simulink model "NoPainNoCrane_Hardware"  (R2016a)
settings: Solver=ode5  StartTime=0.0  StopTime=59.6965  FixedStep=0.01  RelTol=1e-3
model workspace: external: MAT-File workspace.mat (data not in the file)
values from neighbouring files (symbols this model uses):
  AngleDX = 0    [RunHWModel.m]    (also in simSetup.m; workspace.mat)
  AngleDY = AngleDX    (= 0)    [RunHWModel.m]    (also in simSetup.m; workspace.mat)
  AngleIX = 0    [RunHWModel.m]    (also in simSetup.m; workspace.mat)
  AngleIY = AngleIX    (= 0)    [RunHWModel.m]    (also in simSetup.m; workspace.mat)
  AnglePX = 2.0    (= 2)    [RunHWModel.m]    (also in simSetup.m; workspace.mat)
  AnglePY = AnglePX    (= 2)    [RunHWModel.m]    (also in simSetup.m; workspace.mat)
  DC1x = 0.1    [RunHWModel.m]    (also in simSetup.m; workspace.mat)
  DC1y = DC1x    (= 0.1)    [RunHWModel.m]    (also in simSetup.m; workspace.mat)
  IC1x = 0.9    [RunHWModel.m]    (also in simSetup.m; workspace.mat)
  IC1y = IC1x    (= 0.9)    [RunHWModel.m]    (also in simSetup.m; workspace.mat)
  PC1x = 4.7    [RunHWModel.m]    (also in simSetup.m; workspace.mat)
  PC1y = PC1x    (= 4.7)    [RunHWModel.m]    (also in simSetup.m; workspace.mat)
  Ts = 1/20    (= 0.05)    [setup.m]    (also in workspace.mat)
  waypoints = [waypoints is_target]    [path_planning.m]    (also in workspace.mat = [0 1 4 16 20 20 0 2 5 6 10 20 ... (30 elements, 6x5)])
  xRange = [0 0.52]    [workspace.mat]
  yRange = [0 0.62]    [workspace.mat]
undefined symbols (not defined in the file or in its folder): Crane3D_RangeBit, Crane3D_ScaleCoeff
undefined symbols (not defined in the file): RTDAC4PCIBaseAddress
libraries: simulink x4
settings Model: SimulationMode=external  ExtModeTrigDuration=10000  Creator=The MathWorks Inc.  LastModifiedBy=mc1713
settings DataIOCC: SaveFormat=StructureWithTime  SignalLoggingSaveFormat=ModelDataLogs  SignalLoggingName=logsOut
settings OptimizationCC: ExpressionDepthLimit=2147483647  InitFltsAndDblsToZero=on  EfficientMapNaN2IntZero=off
settings DebuggingCC: UnderspecifiedInitializationDetection=Classic  MergeDetectMultiDrivingBlocksExec=none  SignalResolutionControl=TryResolveAllWithWarning  FcnCallInpInsideContextMsg=EnableAllAsWarning  StateNameClashWarn=warning
settings HardwareCC: ProdBitPerLong=64  ProdLargestAtomicFloat=None  ProdHWDeviceType=Intel->x86-64  TargetBitPerLong=64  TargetBitPerPointer=64  TargetIntDivRoundTo=Zero  TargetEndianess=LittleEndian  TargetWordSize=64  TargetHWDeviceType=Intel->x86-64
settings ModelReferenceCC: UpdateModelReferenceTargets=Force  PropagateSignalLabelsOutOfModel=off
settings RTWCC: SystemTargetFile=sldrt.tlc  TemplateMakefile=sldrt.tmf  Description=Simulink Desktop Real-Time  RTWCompilerOptimization=on
settings CodeAppCC: MaxIdLength=95
settings TargetCC: TargetPreCompLibLocation=C:\matlab\R2016a\toolbox\sldrt\lib\win64  GeneratePreprocessorConditionals=Use local settings
settings ConfigComp: CovSFcnEnable=off

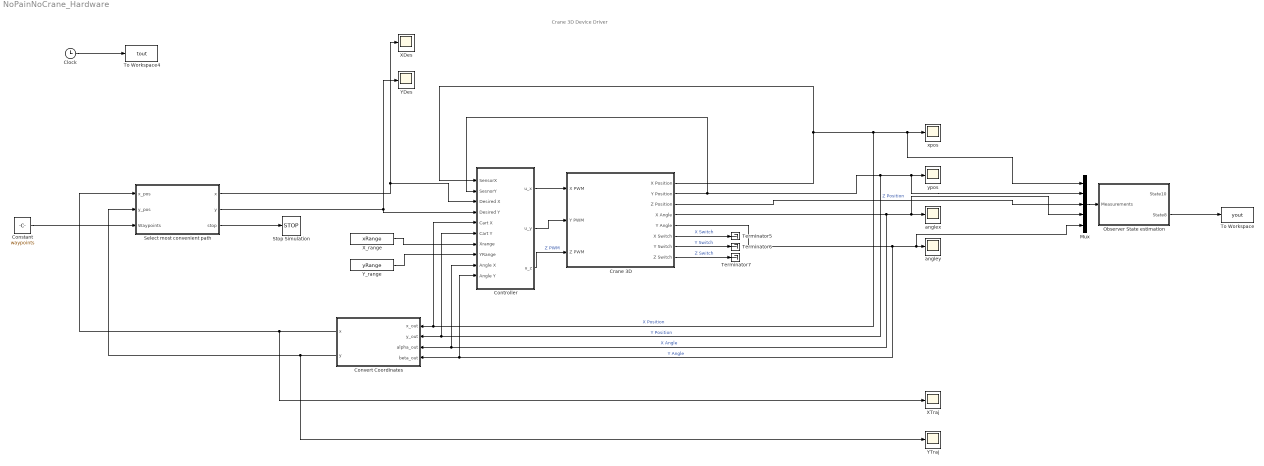
== system NoPainNoCrane_Hardware ==
  note: Crane 3D Device Driver
  Clock : Clock
  Constant : Constant  Value=waypoints
  Controller : Subsystem
  Convert Coordinates : MATLAB Function  TreatAsAtomicUnit=on
  Crane 3D : Subsystem  mask{BaseAddress=RTDAC4PCIBaseAddress, T0=0.01}
      mask prompts: BaseAddress "Base Address:"; T0 "Samping Period:"
      mask Display: image(imread('crane.jpeg'))
  Mux : Mux  Inputs=5
  Observer State estimation : Subsystem
  Select most convenient path : MATLAB Function  TreatAsAtomicUnit=on
  Stop Simulation : Stop
  Terminator5 : Terminator
  Terminator6 : Terminator
  Terminator7 : Terminator
  To Workspace : ToWorkspace  VariableName=yout  SaveFormat=Structure With Time  SampleTime=-1
  To Workspace4 : ToWorkspace  VariableName=tout  SaveFormat=Structure With Time  SampleTime=-1
  XDes : Scope
  XTraj : Scope
  X_range : Constant  Value=xRange
  YDes : Scope
  YTraj : Scope
  "Y_range " : Constant  Value=yRange
  anglex : Scope
  angley : Scope
  xpos : Scope
  ypos : Scope
  wires:
  Crane 3D/6(X Switch) -> Terminator5/1  "X Switch"
  Crane 3D/7(Y Switch) -> Terminator6/1  "Y Switch"
  Crane 3D/8(Z Switch) -> Terminator7/1  "Z Switch"
  Crane 3D/1(X Position) -> Controller/5(Cart X), Convert Coordinates/1(x_out), Mux/1, xpos/1, Controller/1(SensorX)  "X Position"
  Crane 3D/2(Y Position) -> Controller/2(SesnorY), Controller/6(Cart Y), Convert Coordinates/2(y_out), Mux/2, ypos/1  "Y Position"
  Crane 3D/3(Z Position) -> Mux/3  "Z Position"
  Crane 3D/4(X Angle) -> Controller/9(Angle X), Convert Coordinates/3(alpha_out), Mux/4, anglex/1  "X Angle"
  Crane 3D/5(Y Angle) -> Controller/10(Angle Y), Convert Coordinates/4(beta_out), Mux/5, angley/1  "Y Angle"
  Controller/3(u_z) -> Crane 3D/3(Z PWM)  "Z PWM"
  Clock/1 -> To Workspace4/1
  Convert Coordinates/2(y) -> YTraj/1, Select most convenient path/2(y_pos)
  Convert Coordinates/1(x) -> XTraj/1, Select most convenient path/1(x_pos)
  Controller/2(u_y) -> Crane 3D/2(Y PWM)
  Controller/1(u_x) -> Crane 3D/1(X PWM)
  Constant/1 -> Select most convenient path/3(Waypoints)
  Select most convenient path/1(x) -> XDes/1, Controller/3(Desired X)
  Select most convenient path/2(y) -> Controller/4(Desired Y), YDes/1
  X_range/1 -> Controller/7(Xrange)
  "Y_range "/1 -> Controller/8(YRange)
  Select most convenient path/3(stop) -> Stop Simulation/1
  Mux/1 -> Observer State estimation/1(Measurements)
  Observer State estimation/2(State8) -> To Workspace/1

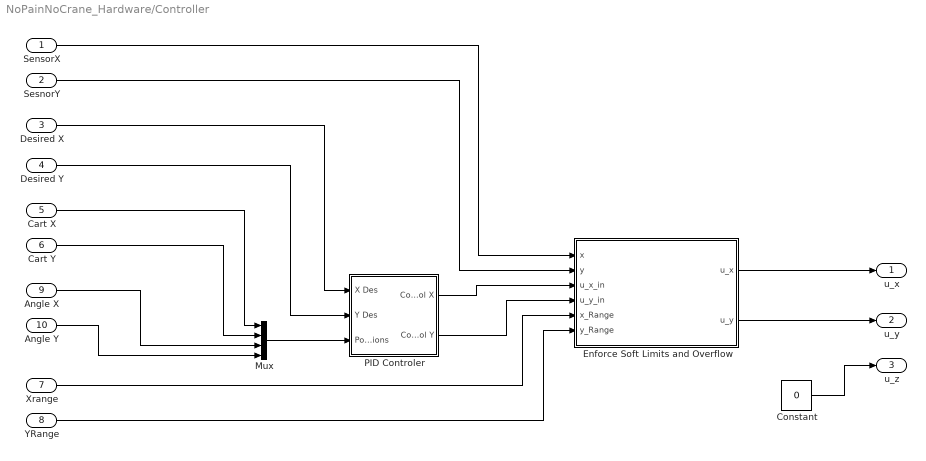
== system NoPainNoCrane_Hardware/Controller ==
  SensorX : Inport
  SesnorY : Inport  Port=2
  Desired X : Inport  Port=3
  Desired Y : Inport  Port=4
  Cart X : Inport  Port=5
  Cart Y : Inport  Port=6
  Xrange : Inport  Port=7
  YRange : Inport  Port=8
  Angle X : Inport  Port=9
  Angle Y : Inport  Port=10
  Constant : Constant  Value=0
  Enforce Soft Limits and Overflow : MATLAB Function  TreatAsAtomicUnit=on
  Mux : Mux
  PID Controler : Subsystem
  u_x : Outport
  u_y : Outport  Port=2
  u_z : Outport  Port=3
  wires:
  Constant/1 -> u_z/1
  Desired X/1 -> PID Controler/1(X Des)
  Desired Y/1 -> PID Controler/2(Y Des)
  Mux/1 -> PID Controler/3(Positions)
  Cart X/1 -> Mux/1
  Cart Y/1 -> Mux/2
  Enforce Soft Limits and Overflow/1(u_x) -> u_x/1
  Enforce Soft Limits and Overflow/2(u_y) -> u_y/1
  PID Controler/1(Control X) -> Enforce Soft Limits and Overflow/3(u_x_in)
  PID Controler/2(Control Y) -> Enforce Soft Limits and Overflow/4(u_y_in)
  Xrange/1 -> Enforce Soft Limits and Overflow/5(x_Range)
  YRange/1 -> Enforce Soft Limits and Overflow/6(y_Range)
  SensorX/1 -> Enforce Soft Limits and Overflow/1(x)
  SesnorY/1 -> Enforce Soft Limits and Overflow/2(y)
  Angle X/1 -> Mux/3
  Angle Y/1 -> Mux/4

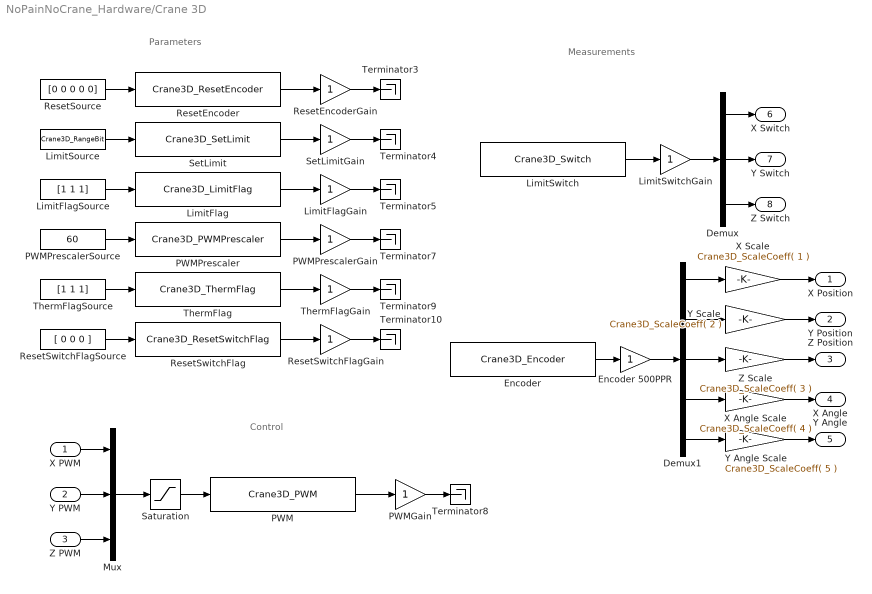
== system NoPainNoCrane_Hardware/Crane 3D ==
  note: Measurements
  note: Control
  note: Parameters
  X PWM : Inport
  Y PWM : Inport  Port=2
  Z PWM : Inport  Port=3
  Demux : Demux  Outputs=3
  Demux1 : Demux  Outputs=5
  Encoder : S-Function  FunctionName=Crane3D_Encoder  Parameters=BaseAddress, T0  SFunctionDeploymentMode=off  EnableBusSupport=off
  Encoder 500PPR : Gain  SaturateOnIntegerOverflow=on  OutDataTypeStr=Inherit: Same as input  ParamDataTypeStr=Inherit: Same as input
  LimitFlag : S-Function  FunctionName=Crane3D_LimitFlag  Parameters=BaseAddress, T0  SFunctionDeploymentMode=off  EnableBusSupport=off
  LimitFlagGain : Gain  SaturateOnIntegerOverflow=on  OutDataTypeStr=Inherit: Same as input  ParamDataTypeStr=Inherit: Same as input
  LimitFlagSource : Constant  Value=[1 1 1]
  LimitSource : Constant  Value=Crane3D_RangeBit
  LimitSwitch : S-Function  FunctionName=Crane3D_Switch  Parameters=BaseAddress, T0  SFunctionDeploymentMode=off  EnableBusSupport=off
  LimitSwitchGain : Gain  SaturateOnIntegerOverflow=on  OutDataTypeStr=Inherit: Same as input  ParamDataTypeStr=Inherit: Same as input
  Mux : Mux  Inputs=3
  PWM : S-Function  FunctionName=Crane3D_PWM  Parameters=BaseAddress, T0  SFunctionDeploymentMode=off  EnableBusSupport=off
  PWMGain : Gain  SaturateOnIntegerOverflow=on  OutDataTypeStr=Inherit: Same as input  ParamDataTypeStr=Inherit: Same as input
  PWMPrescaler : S-Function  FunctionName=Crane3D_PWMPrescaler  Parameters=BaseAddress, T0  SFunctionDeploymentMode=off  EnableBusSupport=off
  PWMPrescalerGain : Gain  SaturateOnIntegerOverflow=on  OutDataTypeStr=Inherit: Same as input  ParamDataTypeStr=Inherit: Same as input
  PWMPrescalerSource : Constant  Value=60
  ResetEncoder : S-Function  FunctionName=Crane3D_ResetEncoder  Parameters=BaseAddress, T0  SFunctionDeploymentMode=off  EnableBusSupport=off
  ResetEncoderGain : Gain  SaturateOnIntegerOverflow=on  OutDataTypeStr=Inherit: Same as input  ParamDataTypeStr=Inherit: Same as input
  ResetSource : Constant  Value=[0 0 0 0 0]
  "ResetSwitchFlag " : S-Function  FunctionName=Crane3D_ResetSwitchFlag  Parameters=BaseAddress, T0  SFunctionDeploymentMode=off  EnableBusSupport=off
  ResetSwitchFlagGain : Gain  SaturateOnIntegerOverflow=on  OutDataTypeStr=Inherit: Same as input  ParamDataTypeStr=Inherit: Same as input
  ResetSwitchFlagSource : Constant  Value=[ 0 0 0 ]
  Saturation : Saturate  UpperLimit=1  LowerLimit=-1
  SetLimit : S-Function  FunctionName=Crane3D_SetLimit  Parameters=BaseAddress, T0  SFunctionDeploymentMode=off  EnableBusSupport=off
  SetLimitGain : Gain  SaturateOnIntegerOverflow=on  OutDataTypeStr=Inherit: Same as input  ParamDataTypeStr=Inherit: Same as input
  Terminator{3..5,7..10} (7 alike) : Terminator
  "ThermFlag " : S-Function  FunctionName=Crane3D_ThermFlag  Parameters=BaseAddress, T0  SFunctionDeploymentMode=off  EnableBusSupport=off
  ThermFlagGain : Gain  SaturateOnIntegerOverflow=on  OutDataTypeStr=Inherit: Same as input  ParamDataTypeStr=Inherit: Same as input
  ThermFlagSource : Constant  Value=[1 1 1]
  X Angle Scale : Gain  Gain=Crane3D_ScaleCoeff( 4 )  OutDataTypeStr=Inherit: Same as input  ParamDataTypeStr=Inherit: Same as input
  X Scale : Gain  Gain=Crane3D_ScaleCoeff( 1 )  OutDataTypeStr=Inherit: Same as input  ParamDataTypeStr=Inherit: Same as input
  Y Angle Scale : Gain  Gain=Crane3D_ScaleCoeff( 5 )  OutDataTypeStr=Inherit: Same as input  ParamDataTypeStr=Inherit: Same as input
  Y Scale : Gain  Gain=Crane3D_ScaleCoeff( 2 )  OutDataTypeStr=Inherit: Same as input  ParamDataTypeStr=Inherit: Same as input
  Z Scale : Gain  Gain=Crane3D_ScaleCoeff( 3 )  OutDataTypeStr=Inherit: Same as input  ParamDataTypeStr=Inherit: Same as input
  X Position : Outport  InitialOutput=0
  Y Position : Outport  Port=2  InitialOutput=0
  Z Position : Outport  Port=3  InitialOutput=0
  X Angle : Outport  Port=4  InitialOutput=0
  Y Angle : Outport  Port=5  InitialOutput=0
  X Switch : Outport  Port=6  InitialOutput=0
  Y Switch : Outport  Port=7  InitialOutput=0
  Z Switch : Outport  Port=8  InitialOutput=0
  wires:
  Demux1/1 -> X Scale/1
  Demux1/2 -> Y Scale/1
  Demux1/3 -> Z Scale/1
  Demux1/4 -> X Angle Scale/1
  Demux1/5 -> Y Angle Scale/1
  X Angle Scale/1 -> X Angle/1
  Y Angle Scale/1 -> Y Angle/1
  Y Scale/1 -> Y Position/1
  X Scale/1 -> X Position/1
  Z Scale/1 -> Z Position/1
  Demux/3 -> Z Switch/1
  Demux/2 -> Y Switch/1
  Demux/1 -> X Switch/1
  LimitSwitchGain/1 -> Demux/1
  LimitSwitch/1 -> LimitSwitchGain/1
  X PWM/1 -> Mux/1
  Y PWM/1 -> Mux/2
  Z PWM/1 -> Mux/3
  ResetSwitchFlagGain/1 -> Terminator10/1
  ThermFlagGain/1 -> Terminator9/1
  PWMPrescalerGain/1 -> Terminator7/1
  LimitFlagGain/1 -> Terminator5/1
  SetLimitGain/1 -> Terminator4/1
  ResetEncoderGain/1 -> Terminator3/1
  ResetSwitchFlagSource/1 -> "ResetSwitchFlag "/1
  ThermFlagSource/1 -> "ThermFlag "/1
  PWMPrescalerSource/1 -> PWMPrescaler/1
  LimitFlagSource/1 -> LimitFlag/1
  LimitSource/1 -> SetLimit/1
  ResetSource/1 -> ResetEncoder/1
  "ResetSwitchFlag "/1 -> ResetSwitchFlagGain/1
  "ThermFlag "/1 -> ThermFlagGain/1
  PWMPrescaler/1 -> PWMPrescalerGain/1
  LimitFlag/1 -> LimitFlagGain/1
  SetLimit/1 -> SetLimitGain/1
  ResetEncoder/1 -> ResetEncoderGain/1
  PWMGain/1 -> Terminator8/1
  PWM/1 -> PWMGain/1
  Mux/1 -> Saturation/1
  Saturation/1 -> PWM/1
  Encoder/1 -> Encoder 500PPR/1
  Encoder 500PPR/1 -> Demux1/1

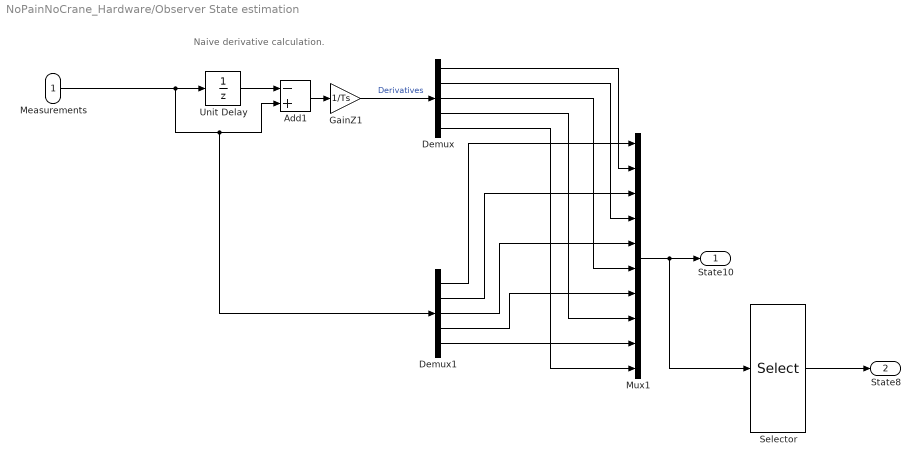
== system NoPainNoCrane_Hardware/Observer State estimation ==
  note: Naive derivative calculation.
  Measurements : Inport
  Add1 : Sum  Inputs=-+
  Demux : Demux  Outputs=5
  Demux1 : Demux  Outputs=5
  GainZ1 : Gain  Gain=1/Ts  SaturateOnIntegerOverflow=on  OutDataTypeStr=Inherit: Same as input  ParamDataTypeStr=Inherit: Same as input
  Mux1 : Mux  Inputs=10
  Selector : Selector  InputPortWidth=10  IndexOptions=Index vector (dialog)  Indices=[1:4 7:10]  OutputSizes=1
  Unit Delay : UnitDelay  InitialCondition="[0.26 0.32 0.3  0 0]"  SampleTime=-1
  State10 : Outport
  State8 : Outport  Port=2
  wires:
  Unit Delay/1 -> Add1/1
  Add1/1 -> GainZ1/1
  Measurements/1 -> Demux1/1, Add1/2, Unit Delay/1
  GainZ1/1 -> Demux/1  "Derivatives"
  Mux1/1 -> Selector/1, State10/1
  Demux1/1 -> Mux1/1
  Demux/1 -> Mux1/2
  Demux1/2 -> Mux1/3
  Demux1/3 -> Mux1/5
  Demux1/4 -> Mux1/7
  Demux1/5 -> Mux1/9
  Demux/2 -> Mux1/4
  Demux/3 -> Mux1/6
  Demux/4 -> Mux1/8
  Demux/5 -> Mux1/10
  Selector/1 -> State8/1

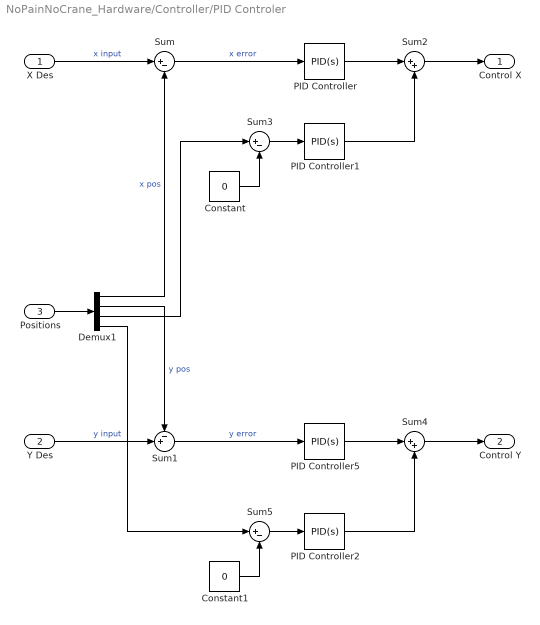
== system NoPainNoCrane_Hardware/Controller/PID Controler ==
  X Des : Inport
  Y Des : Inport  Port=2
  Positions : Inport  Port=3
  Constant : Constant  Value=0
  Constant1 : Constant  Value=0
  Demux1 : Demux
  PID Controller : simulink/Continuous/PID Controller  Controller=PID  TimeDomain=Continuous-time  SampleTime=-1  IntegratorMethod=Forward Euler  FilterMethod=Forward Euler  Form=Parallel  UseFilter=on  ControllerParametersSource=internal  P=PC1x  I=IC1x  D=DC1x  N=30  InitialConditionSource=internal  InitialConditionForIntegrator=0  InitialConditionForFilter=0  ExternalReset=none  LimitOutput=off  UpperSaturationLimit=inf  LowerSaturationLimit=-inf  LinearizeAsGain=on  AntiWindupMode=none  Kb=1  TrackingMode=off  Kt=1  PParamMin=[]  PParamMax=[]  IParamMin=[]  IParamMax=[]  DParamMin=[]  DParamMax=[]  NParamMin=[]  NParamMax=[]  KbParamMin=[]  KbParamMax=[]  KtParamMin=[]  KtParamMax=[]  POutMin=[]  POutMax=[]  IOutMin=[]  IOutMax=[]  DOutMin=[]  DOutMax=[]  NOutMin=[]  NOutMax=[]  KbOutMin=[]  KbOutMax=[]  KtOutMin=[]  KtOutMax=[]  IntegratorOutMin=[]  IntegratorOutMax=[]  FilterOutMin=[]  FilterOutMax=[]  SumOutMin=[]  SumOutMax=[]  SumI1OutMin=[]  SumI1OutMax=[]  SumI2OutMin=[]  SumI2OutMax=[]  SumI3OutMin=[]  SumI3OutMax=[]  SumDOutMin=[]  SumDOutMax=[]  SaturationOutMin=[]  SaturationOutMax=[]  IntegratorContinuousStateAttributes=''  IntegratorStateMustResolveToSignalObject=off  IntegratorRTWStateStorageClass=Auto  FilterContinuousStateAttributes=''  FilterStateMustResolveToSignalObject=off  FilterRTWStateStorageClass=Auto  DifferentiatorICPrevScaledInput=0  DifferentiatorOutMin=[]  DifferentiatorOutMax=[]
  PID Controller1 : simulink/Continuous/PID Controller  Controller=PID  TimeDomain=Continuous-time  SampleTime=-1  IntegratorMethod=Forward Euler  FilterMethod=Forward Euler  Form=Parallel  UseFilter=on  ControllerParametersSource=internal  P=AnglePX  I=AngleIX  D=AngleDX  N=30  InitialConditionSource=internal  InitialConditionForIntegrator=0  InitialConditionForFilter=0  ExternalReset=none  LimitOutput=off  UpperSaturationLimit=inf  LowerSaturationLimit=-inf  LinearizeAsGain=on  AntiWindupMode=none  Kb=1  TrackingMode=off  Kt=1  PParamMin=[]  PParamMax=[]  IParamMin=[]  IParamMax=[]  DParamMin=[]  DParamMax=[]  NParamMin=[]  NParamMax=[]  KbParamMin=[]  KbParamMax=[]  KtParamMin=[]  KtParamMax=[]  POutMin=[]  POutMax=[]  IOutMin=[]  IOutMax=[]  DOutMin=[]  DOutMax=[]  NOutMin=[]  NOutMax=[]  KbOutMin=[]  KbOutMax=[]  KtOutMin=[]  KtOutMax=[]  IntegratorOutMin=[]  IntegratorOutMax=[]  FilterOutMin=[]  FilterOutMax=[]  SumOutMin=[]  SumOutMax=[]  SumI1OutMin=[]  SumI1OutMax=[]  SumI2OutMin=[]  SumI2OutMax=[]  SumI3OutMin=[]  SumI3OutMax=[]  SumDOutMin=[]  SumDOutMax=[]  SaturationOutMin=[]  SaturationOutMax=[]  IntegratorContinuousStateAttributes=''  IntegratorStateMustResolveToSignalObject=off  IntegratorRTWStateStorageClass=Auto  FilterContinuousStateAttributes=''  FilterStateMustResolveToSignalObject=off  FilterRTWStateStorageClass=Auto  DifferentiatorICPrevScaledInput=0  DifferentiatorOutMin=[]  DifferentiatorOutMax=[]
  PID Controller2 : simulink/Continuous/PID Controller  Controller=PID  TimeDomain=Continuous-time  SampleTime=-1  IntegratorMethod=Forward Euler  FilterMethod=Forward Euler  Form=Parallel  UseFilter=on  ControllerParametersSource=internal  P=AnglePY  I=AngleIY  D=AngleDY  N=30  InitialConditionSource=internal  InitialConditionForIntegrator=0  InitialConditionForFilter=0  ExternalReset=none  LimitOutput=off  UpperSaturationLimit=inf  LowerSaturationLimit=-inf  LinearizeAsGain=on  AntiWindupMode=none  Kb=1  TrackingMode=off  Kt=1  PParamMin=[]  PParamMax=[]  IParamMin=[]  IParamMax=[]  DParamMin=[]  DParamMax=[]  NParamMin=[]  NParamMax=[]  KbParamMin=[]  KbParamMax=[]  KtParamMin=[]  KtParamMax=[]  POutMin=[]  POutMax=[]  IOutMin=[]  IOutMax=[]  DOutMin=[]  DOutMax=[]  NOutMin=[]  NOutMax=[]  KbOutMin=[]  KbOutMax=[]  KtOutMin=[]  KtOutMax=[]  IntegratorOutMin=[]  IntegratorOutMax=[]  FilterOutMin=[]  FilterOutMax=[]  SumOutMin=[]  SumOutMax=[]  SumI1OutMin=[]  SumI1OutMax=[]  SumI2OutMin=[]  SumI2OutMax=[]  SumI3OutMin=[]  SumI3OutMax=[]  SumDOutMin=[]  SumDOutMax=[]  SaturationOutMin=[]  SaturationOutMax=[]  IntegratorContinuousStateAttributes=''  IntegratorStateMustResolveToSignalObject=off  IntegratorRTWStateStorageClass=Auto  FilterContinuousStateAttributes=''  FilterStateMustResolveToSignalObject=off  FilterRTWStateStorageClass=Auto  DifferentiatorICPrevScaledInput=0  DifferentiatorOutMin=[]  DifferentiatorOutMax=[]
  PID Controller5 : simulink/Continuous/PID Controller  Controller=PID  TimeDomain=Continuous-time  SampleTime=-1  IntegratorMethod=Forward Euler  FilterMethod=Forward Euler  Form=Parallel  UseFilter=on  ControllerParametersSource=internal  P=PC1y  I=IC1y  D=DC1y  N=30  InitialConditionSource=internal  InitialConditionForIntegrator=0  InitialConditionForFilter=0  ExternalReset=none  LimitOutput=off  UpperSaturationLimit=inf  LowerSaturationLimit=-inf  LinearizeAsGain=on  AntiWindupMode=none  Kb=1  TrackingMode=off  Kt=1  PParamMin=[]  PParamMax=[]  IParamMin=[]  IParamMax=[]  DParamMin=[]  DParamMax=[]  NParamMin=[]  NParamMax=[]  KbParamMin=[]  KbParamMax=[]  KtParamMin=[]  KtParamMax=[]  POutMin=[]  POutMax=[]  IOutMin=[]  IOutMax=[]  DOutMin=[]  DOutMax=[]  NOutMin=[]  NOutMax=[]  KbOutMin=[]  KbOutMax=[]  KtOutMin=[]  KtOutMax=[]  IntegratorOutMin=[]  IntegratorOutMax=[]  FilterOutMin=[]  FilterOutMax=[]  SumOutMin=[]  SumOutMax=[]  SumI1OutMin=[]  SumI1OutMax=[]  SumI2OutMin=[]  SumI2OutMax=[]  SumI3OutMin=[]  SumI3OutMax=[]  SumDOutMin=[]  SumDOutMax=[]  SaturationOutMin=[]  SaturationOutMax=[]  IntegratorContinuousStateAttributes=''  IntegratorStateMustResolveToSignalObject=off  IntegratorRTWStateStorageClass=Auto  FilterContinuousStateAttributes=''  FilterStateMustResolveToSignalObject=off  FilterRTWStateStorageClass=Auto  DifferentiatorICPrevScaledInput=0  DifferentiatorOutMin=[]  DifferentiatorOutMax=[]
  Sum : Sum  Inputs=|+-
  Sum1 : Sum  Inputs=-+|
  Sum2 : Sum  Inputs=|++
  Sum3 : Sum  Inputs=|+-
  Sum4 : Sum  Inputs=|++
  Sum5 : Sum  Inputs=|+-
  Control X : Outport
  Control Y : Outport  Port=2
  wires:
  Demux1/1 -> Sum/2  "x pos"
  X Des/1 -> Sum/1  "x input"
  Sum/1 -> PID Controller/1  "x error"
  Demux1/2 -> Sum1/1  "y pos"
  Y Des/1 -> Sum1/2  "y input"
  Positions/1 -> Demux1/1
  Sum1/1 -> PID Controller5/1  "y error"
  PID Controller/1 -> Sum2/1
  PID Controller1/1 -> Sum2/2
  Sum3/1 -> PID Controller1/1
  Demux1/3 -> Sum3/1
  Constant/1 -> Sum3/2
  Sum2/1 -> Control X/1
  PID Controller5/1 -> Sum4/1
  Sum4/1 -> Control Y/1
  PID Controller2/1 -> Sum4/2
  Sum5/1 -> PID Controller2/1
  Constant1/1 -> Sum5/2
  Demux1/4 -> Sum5/1

== matlab function NoPainNoCrane_Hardware/Controller/Enforce Soft Limits and Overflow ==
  data: x input; u_x output; y input; u_x_in input; u_y_in input; x_Range input; y_Range input; u_y output
function [u_x, u_y] = fcn(x, y, u_x_in, u_y_in, x_Range, y_Range)

buff_up = 0.08;
buff_low = 0.08;
u_x = u_x_in;
u_y = u_y_in;

% Deal with overflow - may not be the most appropriate place
if(x > 10 || x < -10)
   x = 0;
end
if (y > 10 || y < -10)
   y = 0;
end

% Put in place soft boundaries on the borders
if (x > (x_Range(2)-buff_up))
    u_x = min(u_x_in,0);
end

if (x < (x_Range(1)+buff_low))
    u_x = max(u_x_in,0);
end


if (y > (y_Range(2)-buff_up))
    u_y = min(u_y_in,0);
end

if (y < (y_Range(1)+buff_low))
    u_y = max(u_y_in,0);
end


end

== matlab function NoPainNoCrane_Hardware/Select most convenient path ==
  data: x output; y output; x_pos input; y_pos input; Waypoints input; stop output
function [x,y, stop] = Path_Selector(x_pos, y_pos, Waypoints)
persistent WP_Index

if isempty(WP_Index)
    WP_Index = 1;
end

%% Random default values - dont touch
x = 0.252;
y = 0.365;
stop = 0;
if WP_Index <= (length(Waypoints))
    x = Waypoints(WP_Index,1)/100;
    y = Waypoints(WP_Index,2)/100;
    
    %% Establish boundary conditions and controller class
    x_max = x+0.02;
    x_min = x-0.02;
    y_max = y+0.02;
    y_min = y-0.02;
    
    if Waypoints(WP_Index,5) == 1
        x_max = x+0.01;
        x_min = x-0.01;
        y_max = y+0.01;
        y_min = y-0.01;
    end
    
    
    %% Crane arrived to point
    if (((x_pos <= x_max) && (x_pos >= x_min)) && ((y_pos <= y_max) && (y_pos >= y_min)))
        WP_Index = WP_Index + 1; 
        if WP_Index > (length(Waypoints))
            WP_Index = WP_Index - 1;
            stop = 1
        end
    end
end

== matlab function NoPainNoCrane_Hardware/Convert Coordinates ==
  data: x output; y output; x_out input; y_out input; alpha_out input; beta_out input
function [x,y] = Sensors2World(x_out,y_out,alpha_out, beta_out)

%% Assumptions
R = 0.3;

%% Obtain Measurements from sensors
now_x = x_out;
now_y = y_out;
now_alpha = alpha_out;
now_beta = beta_out;

sin_a = sin(now_alpha);
sin_b = sin(now_beta);
cos_a = cos(now_alpha);

% x = now_x + R * sin_a * sin_b;
% y = now_y + R * cos_a;

x = now_x + R * sin_a;
y = now_y + R * sin_b;
